simulink model "testTorqueFree"  (R2021a)
settings: Solver=VariableStepAuto  StartTime=0.0  StopTime=Torb  RelTol=1e-3
libraries: sharedtransform x1
settings Model: DataDictionary=databus.sldd  Creator=Laura  LastModifiedBy=Laura

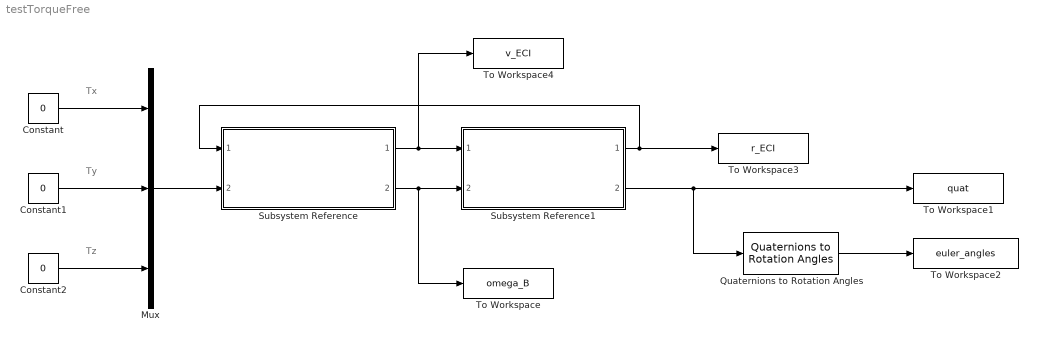
== system testTorqueFree ==
  note: Tx
  note: Ty
  note: Tz
  Constant : Constant  Value=0
  Constant1 : Constant  Value=0
  Constant2 : Constant  Value=0
  Mux : Mux  Inputs=3
  Quaternions to Rotation Angles : sharedtransform/Quaternions to Rotation Angles  rotationOrder=ZYX  aMode=aMode
      settings: SourceProductBaseCode=AE,PW,DR,MT,UV,VE
  Subsystem Reference : Subsystem  ReferencedSubsystem=Dynamics
  Subsystem Reference1 : Subsystem  ReferencedSubsystem=Kinematics
  To Workspace : ToWorkspace  VariableName=omega_B  SaveFormat=Timeseries  SampleTime=-1
  To Workspace1 : ToWorkspace  VariableName=quat  SaveFormat=Timeseries  SampleTime=-1
  To Workspace2 : ToWorkspace  VariableName=euler_angles  SaveFormat=Timeseries  SampleTime=-1
  To Workspace3 : ToWorkspace  VariableName=r_ECI  SaveFormat=Timeseries  SampleTime=-1
  To Workspace4 : ToWorkspace  VariableName=v_ECI  SaveFormat=Timeseries  SampleTime=-1
  wires:
  Quaternions to Rotation Angles/1 -> To Workspace2/1
  Mux/1 -> Subsystem Reference/2
  Subsystem Reference1/1 -> To Workspace3/1, Subsystem Reference/1
  Subsystem Reference1/2 -> To Workspace1/1, Quaternions to Rotation Angles/1
  Subsystem Reference/2 -> To Workspace/1, Subsystem Reference1/2
  Constant1/1 -> Mux/2
  Subsystem Reference/1 -> To Workspace4/1, Subsystem Reference1/1
  Constant2/1 -> Mux/3
  Constant/1 -> Mux/1
